simulink model "TailSitter_PX4"  (R2018b)
settings: Solver=VariableStepAuto  StartTime=0.0  StopTime=1100  RelTol=1e-3
values from neighbouring files (symbols this model uses):
  p =     [ds.mat]    (also in vxs.mat)
undefined symbols (not defined in the file or in its folder): quatnormalize
libraries: aerolibutil x24, simulink x14, sharedtransform x6, vrlib x4, sharedutil x3, simulink_extras x2, aerolibanim x1, aerolibanimutils x1
(part 3 of 3)

== matlab function TailSitter_PX4/AdHoc2 ==
  data: u_jointT input; u_omegaL output; u_omegaR output; u_deltaL output; u_deltaR output; tx input; ty input; tz input
function [u_omegaL,u_omegaR, u_deltaL,u_deltaR]  = AdHocTorques( u_jointT, tx, ty, tz)

% This is a crude/simple input/output/actuator linker.
% A pitch torque is made by moving elevons in the same direction: jointA.
% A roll torque is made by moving elevons in opposite direction: deltaA.
% A yaw torque is made by a differential thrust of the engines: deltaT.
% Power forward is given and passed straight through this function as
% jointT.

u_deltaL = 0;
u_deltaR = 0;
u_omegaL = 0;
u_omegaR = 0;



u_deltaA = -tx;
u_jointA = -ty;
u_deltaT = -tz;

u_deltaL = u_jointA - u_deltaA/2;
u_deltaR = u_jointA + u_deltaA/2;
u_omegaL = u_jointT + u_deltaT/2;
u_omegaR = u_jointT - u_deltaT/2;


end

== matlab function TailSitter_PX4/MATLAB Function3 ==
  data: v_wf input; yaw output; vr_wf input
function yaw = fcn(v_wf, vr_wf)

yawr = atan2(vr_wf(2),vr_wf(1));

if abs(atan2(sqrt(sum(v_wf(1:2).^2)),abs(v_wf(3)))) < 0.1
    yaw = yawr;
else
    yaw = atan2(v_wf(2),v_wf(1));
end

== matlab function TailSitter_PX4/TorqueTranslator ==
  data: u_jointT input; states input; wdots input; pitchoffset input; p parameter; u_omegaL output; u_omegaR output; u_deltaL output; u_deltaR output; equivalent_gains output size=[1,3]
function [u_omegaL, u_omegaR, u_deltaL, u_deltaR, equivalent_gains] = torqueConverter(u_jointT,states, wdots, pitchoffset, p)

% The reference coming in is for angular accelleration, so don't treat it
% as pure torque:
% I*wdot = tao 

%wxr = taos(1)./p.Ix; 
%wyr = taos(2)./p.Iy;
%wzr = taos(3)./p.Iz;

tx = wdots(1)*p.Ix;
ty = wdots(2)*p.Iy;
tz = wdots(3)*p.Iz;
v = states(1:3);
vx = v(1);
vy = v(2);
vz = v(3);

omegaL = states(13);
omegaR = states(14);

%init outputs
u_deltaL = 0;
u_deltaR = 0;
u_omegaL = 0;
u_omegaR = 0;


% We assume propellers always spin one way. Never reverse.
% We know wanted torque, i.e. we know wdot*Iz=taoz=p.yt*(TL-TR)=p.yt*dT
% taoz./p.yt = TL-TR = p.K_T*(omegaL^2-omegaR^2)
% taoz/(p.yt*p.K_T) = omegaL^2-omegaR^2
% we also know
%TL = JT+dT/2
%TR = JT-dt/2
% => TL-TR = dT = taoz
% if TL=p.K_T*omegaL^2 then
%omegaL=sqrt(TL/p.K_T) =>
%omegaL=sqrt( (JT+dt/2)/p.K_T )
u_omegaL2 = (u_jointT+(tz/p.yt)/2)/p.K_T ; % THese share the jointT, half each.
u_omegaR2 =  (u_jointT-(tz/p.yt)/2)/p.K_T ;
if u_omegaL2 < 0
    u_omegaL = 0;
else
    u_omegaL = sqrt(u_omegaL2);
end
if u_omegaR2 < 0
    u_omegaR = 0;
else
    u_omegaR = sqrt(u_omegaR2);
end

% Lets make a few (crude) approximations.
% - Damping due to rotational speed doesn't exist.
% - Winglets have no z-offset.
% - Wings provide no pitch moment from lift
% Then we come to these formulas for torque around each axis:
%f1 = p.yf.*(FLT+FL -FRT-FR)
%f2 = p.xf.*(FLT+FL+FRT+FR) ...
%f3 = p.yt.*(TL-TR) ...
% 
% They essentially say that aileroins are effective proportioanlly to the
% (square) of the air velocity over them.
% Lets invert that and use as our tunable gain.

% airflow in thrust wake
v_w_L = p.b_w .* omegaL; %[b_w .* omegaL; vy; vz];
v_w_R = p.b_w .* omegaR;
% AILERONS
% Lift inside wake, signs bc rotation dir of aileron
%dFT = -p.CLdelta * 0.5*p.rho * p.Saw;% * deltaL*v_w_L.^2;
 dFT = -p.CLdelta * 0.5*p.rho * p.Saw;% * deltaR*v_w_R.^2;
% Lift outside wake
dF = -sign(vx).*p.CLdelta * 0.5*p.rho*(vx.^2 + vy.^2 + vz.^2) * p.Sa;% * deltaL;

%taoy = p.xf.*(FLT+FL+FRT+FR) ...
%taoy/p.xf = FLT+FL+FRT+FR
%taoy/p.xf = dFT*deltaL*v_w_L.^2 + dFT*deltaR*v_w_R.^2 +dF*(deltaL+deltaR);
%taoy/p.xf = dFT*jointA*v_w_L.^2 + dFT*jointA*v_w_R.^2 +dF*(2*jointA);
%taoy/p.xf = jointA(dFT*v_w_L.^2 + dFT*v_w_R.^2 +dF*2);
%taoy/(p.xf*(dFT*v_w_L.^2 + dFT*v_w_R.^2 +dF*2)) = jointA;
%%%u_jointA = ty/(p.xf*(dFT*v_w_L.^2 + dFT*v_w_R.^2 +dF*2));


%taox/p.yf = (dFLT+dFL)*deltaL - (dFRT+dFR)*deltaR;
%taox/p.yf = dF(deltaL-deltaR) + dFLT*deltaL -dFRT*deltaR;
%toax/p.yf = dF(deltaL-deltaR) + dFT*(deltaL*v_w_L.^2 - deltaR*v_w_R.^2)
%toax/p.yf = -dF*dA + dFT*(deltaL*v_w_L.^2 - deltaR*v_w_R.^2)

%deltaL = JA - dA/2; % Probably bad assumption, jump to other assumptiom
%deltaR = JA + dA/2; => 
%toax/p.yf = -dF*dA + dFT*((JA-dA/2)*v_w_L.^2 - (JA+dA/2)*v_w_R.^2)
%toax/p.yf = -dF*dA + dFT*( JA*v_w_L.^2 - dA*v_w_L.^2/2 - JA*v_w_R.^2 + dA*v_w_R.^2/2)
%toax/p.yf = -dF*dA + dFT*JA(v_w_L.^2-v_w_R.^2) - ( dA*v_w_L.^2/2  - dA*v_w_R.^2/2)
%toax/p.yf - dFT*JA(v_w_L.^2-v_w_R.^2) = -dF*dA - dA*(v_w_L.^2 -v_w_R.^2)/2
%toax/p.yf - dFT*JA(v_w_L.^2-v_w_R.^2) = -dA(dF + (v_w_L.^2 -v_w_R.^2)/2)
%-(toax/p.yf - dFT*JA(v_w_L.^2-v_w_R.^2)) / (dF + (v_w_L.^2 -v_w_R.^2)/2) = dA
%u_deltaA = -(tx/p.yf - dFT*u_jointA*(v_w_L.^2-v_w_R.^2)) / (dF + (v_w_L.^2 -v_w_R.^2)/2);

%taox/p.yf = (dFLT+dFL)*deltaL - (dFRT+dFR)*deltaR;
%taox/p.yf = dF(deltaL-deltaR) + dFLT*deltaL -dFRT*deltaR;
%toax/p.yf = dF(deltaL-deltaR) + dFT*(deltaL*v_w_L.^2 - deltaR*v_w_R.^2)
%toax/p.yf = -dF*dA + dFT*(deltaL*v_w_L.^2 - deltaR*v_w_R.^2)

%deltaL = -dA/2; % Maube correct assumption?
%deltaR = +dA/2; => 
%toax/p.yf = -dF*dA + dFT*((-dA/2)*v_w_L.^2 - (+dA/2)*v_w_R.^2)
%toax/p.yf = -dF*dA + dFT*( - dA*v_w_L.^2/2   dA*v_w_R.^2/2)
%toax/p.yf = -dF*dA - ( dA*v_w_L.^2/2  - dA*v_w_R.^2/2)
%toax/p.yf = -dF*dA - dA*(v_w_L.^2 -v_w_R.^2)/2
%toax/p.yf = -dA(dF + (v_w_L.^2 -v_w_R.^2)/2)
%-(toax/p.yf) / (dF + (v_w_L.^2 -v_w_R.^2)/2) = dA
%%%u_deltaA = -(tx/p.yf) / (dF + 0*0.5*(v_w_L.^2 -v_w_R.^2));


%u_deltaA = (365.0*(3.66e97*omegaL^2*tx + 3.66e97*omegaR^2*tx - 6.17e97*omegaL^2*ty + 6.17e97*omegaR^2*ty - 1.32e91*omegaL^3*abs(omegaL) + 1.32e91*omegaR^3*abs(omegaR) - 2.53e94*omegaL^2*vx*(vx^2 + vz^2)^(1/2) + 2.53e94*omegaR^2*vx*(vx^2 + vz^2)^(1/2) - 2.59e95*omegaL^2*vz*(vx^2 + vz^2)^(1/2) + 2.59e95*omegaR^2*vz*(vx^2 + vz^2)^(1/2) + 1.32e91*omegaL*omegaR^2*abs(omegaL) - 1.32e91*omegaL^2*omegaR*abs(omegaR) + 6.36e100*tx*vx^2*sign(vx) + 6.36e100*tx*vy^2*sign(vx) + 6.36e100*tx*vz^2*sign(vx) + 2.53e95*omegaL^2*vz*cos(2.0*atan2(1.0*vz, vx))*(vx^2 + vz^2)^(1/2) - 2.53e95*omegaR^2*vz*cos(2.0*atan2(1.0*vz, vx))*(vx^2 + vz^2)^(1/2) - 1.52e95*omegaL^2*vx*sin(2.0*atan2(1.0*vz, vx))*(vx^2 + vz^2)^(1/2) + 1.52e95*omegaR^2*vx*sin(2.0*atan2(1.0*vz, vx))*(vx^2 + vz^2)^(1/2)))/(8.21e100*vx^4*sign(vx)^2 + 8.21e100*vy^4*sign(vx)^2 + 8.21e100*vz^4*sign(vx)^2 + 1.09e95*omegaL^2*omegaR^2 + 1.64e101*vx^2*vy^2*sign(vx)^2 + 1.64e101*vx^2*vz^2*sign(vx)^2 + 1.64e101*vy^2*vz^2*sign(vx)^2 + 9.45e97*omegaL^2*vx^2*sign(vx) + 9.45e97*omegaR^2*vx^2*sign(vx) + 9.45e97*omegaL^2*vy^2*sign(vx) + 9.45e97*omegaR^2*vy^2*sign(vx) + 9.45e97*omegaL^2*vz^2*sign(vx) + 9.45e97*omegaR^2*vz^2*sign(vx));
%u_jointA = -(1.46*(4.58e99*omegaR^2*tx - 4.58e99*omegaL^2*tx + 7.71e99*omegaL^2*ty + 7.71e99*omegaR^2*ty + 1.64e93*omegaL^3*abs(omegaL) + 1.64e93*omegaR^3*abs(omegaR) + 3.16e96*omegaL^2*vx*(vx^2 + vz^2)^(1/2) + 3.16e96*omegaR^2*vx*(vx^2 + vz^2)^(1/2) + 3.24e97*omegaL^2*vz*(vx^2 + vz^2)^(1/2) + 3.24e97*omegaR^2*vz*(vx^2 + vz^2)^(1/2) + 1.64e93*omegaL*omegaR^2*abs(omegaL) + 1.64e93*omegaL^2*omegaR*abs(omegaR) + 5.49e99*vx^3*sign(vx)*(vx^2 + vz^2)^(1/2) + 5.63e100*vz^3*sign(vx)*(vx^2 + vz^2)^(1/2) + 1.34e103*ty*vx^2*sign(vx) + 1.34e103*ty*vy^2*sign(vx) + 1.34e103*ty*vz^2*sign(vx) + 5.49e99*vx*vy^2*sign(vx)*(vx^2 + vz^2)^(1/2) + 5.49e99*vx*vz^2*sign(vx)*(vx^2 + vz^2)^(1/2) + 5.63e100*vx^2*vz*sign(vx)*(vx^2 + vz^2)^(1/2) + 5.63e100*vy^2*vz*sign(vx)*(vx^2 + vz^2)^(1/2) + 2.86e96*omegaL*vx^2*abs(omegaL)*sign(vx) + 2.86e96*omegaR*vx^2*abs(omegaR)*sign(vx) + 2.86e96*omegaL*vy^2*abs(omegaL)*sign(vx) + 2.86e96*omegaR*vy^2*abs(omegaR)*sign(vx) + 2.86e96*omegaL*vz^2*abs(omegaL)*sign(vx) + 2.86e96*omegaR*vz^2*abs(omegaR)*sign(vx) - 3.16e97*omegaL^2*vz*cos(2.0*atan2(1.0*vz, vx))*(vx^2 + vz^2)^(1/2) - 3.16e97*omegaR^2*vz*cos(2.0*atan2(1.0*vz, vx))*(vx^2 + vz^2)^(1/2) + 1.9e97*omegaL^2*vx*sin(2.0*atan2(1.0*vz, vx))*(vx^2 + vz^2)^(1/2) + 1.9e97*omegaR^2*vx*sin(2.0*atan2(1.0*vz, vx))*(vx^2 + vz^2)^(1/2) - 5.49e100*vz^3*cos(2.0*atan2(1.0*vz, vx))*sign(vx)*(vx^2 + vz^2)^(1/2) + 3.29e100*vx^3*sin(2.0*atan2(1.0*vz, vx))*sign(vx)*(vx^2 + vz^2)^(1/2) - 5.49e100*vx^2*vz*cos(2.0*atan2(1.0*vz, vx))*sign(vx)*(vx^2 + vz^2)^(1/2) - 5.49e100*vy^2*vz*cos(2.0*atan2(1.0*vz, vx))*sign(vx)*(vx^2 + vz^2)^(1/2) + 3.29e100*vx*vy^2*sin(2.0*atan2(1.0*vz, vx))*sign(vx)*(vx^2 + vz^2)^(1/2) + 3.29e100*vx*vz^2*sin(2.0*atan2(1.0*vz, vx))*sign(vx)*(vx^2 + vz^2)^(1/2)))/(8.21e100*vx^4*sign(vx)^2 + 8.21e100*vy^4*sign(vx)^2 + 8.21e100*vz^4*sign(vx)^2 + 1.09e95*omegaL^2*omegaR^2 + 1.64e101*vx^2*vy^2*sign(vx)^2 + 1.64e101*vx^2*vz^2*sign(vx)^2 + 1.64e101*vy^2*vz^2*sign(vx)^2 + 9.45e97*omegaL^2*vx^2*sign(vx) + 9.45e97*omegaR^2*vx^2*sign(vx) + 9.45e97*omegaL^2*vy^2*sign(vx) + 9.45e97*omegaR^2*vy^2*sign(vx) + 9.45e97*omegaL^2*vz^2*sign(vx) + 9.45e97*omegaR^2*vz^2*sign(vx));


%u_deltaL = u_jointA - u_deltaA/2;
%u_deltaR = u_jointA + u_deltaA/2;

% Below includes pitch down moment from lift
%u_deltaL = -(1.0*(0.5*ty - 0.00102*(vx^2 + vz^2)^(1/2)*(vz*(2.0*cos(2.0*atan2(1.0*vz, vx)) - 2.05) - 1.0*vx*(1.2*sin(2.0*atan2(1.0*vz, vx)) + 0.2)) + 2.13e-7*omegaL*abs(omegaL)))/(0.00209*sign(vx)*(vx^2 + vy^2 + vz^2) + 2.41e-6*omegaL^2) - (0.5*tx)/(0.00353*sign(vx)*(vx^2 + vy^2 + vz^2) + 4.06e-6*omegaL^2);
%u_deltaR =  (0.5*tx)/(0.00353*sign(vx)*(vx^2 + vy^2 + vz^2) + 4.06e-6*omegaR^2) - (1.0*(0.5*ty - 0.00102*(vx^2 + vz^2)^(1/2)*(vz*(2.0*cos(2.0*atan2(1.0*vz, vx)) - 2.05) - 1.0*vx*(1.2*sin(2.0*atan2(1.0*vz, vx)) + 0.2)) + 2.13e-7*omegaR*abs(omegaR)))/(0.00209*sign(vx)*(vx^2 + vy^2 + vz^2) + 2.41e-6*omegaR^2);

% Below only includes sensitivity from airflow % The pitch offet is our
% mechanical trim on the aircraft.
v2 = (vx^2 + vy^2 + vz^2);
omegaL_f = omegaL; %omegas_filt(1);
omegaR_f = omegaR; %omegas_filt(2);
u_deltaL = -(0.5*ty) / (0.00209*sign(vx)*v2 + 2.41e-6*omegaL_f.^2) - (0.5*tx) / (0.00353*sign(vx)*v2 + 4.06e-6*omegaL_f.^2) + pitchoffset;
u_deltaR =  (0.5*tx) / (0.00353*sign(vx)*v2 + 4.06e-6*omegaR_f.^2) - (0.5*ty) / (0.00209*sign(vx)*v2 + 2.41e-6*omegaR_f.^2) + pitchoffset;
 

% The equivalent gains are very misleading, so don't use them much.
equivalent_gains = [ (u_deltaL-u_deltaR)./tx, 0.5*(u_deltaL+u_deltaR)./ty, ...
    (u_omegaL-u_omegaR)./tz];

== matlab function TailSitter_PX4/MATLAB Function5 ==
  data: angErr input; taos output; w input; hovermode input
function taos = fcn(angErr, w, hovermode)

taos = [0;0;0];

P1_fly = 4;
P2_fly = 1.5;
cx_fly = -1;
cy_fly = 1;
cz_fly = -30;

P1_hover = 4;
P2_hover = 2.5-0.5;
cx_hover = -0.6/20;
cy_hover =  0.6;
cz_hover = -120;

if hovermode
    % Emil Fresk P2 controller
    taos = -P1_hover.*angErr - P2_hover.*w;
    % Adjustment for actuators
    taos(1) = cx_hover*taos(1);
    taos(2) = cy_hover*taos(2);
    taos(3) = cz_hover*taos(3);
else
    taos = -P1_fly.*angErr - P2_fly.*w;
    taos(1) = cx_fly*taos(1);
    taos(2) = cy_fly*taos(2);
    taos(3) = cz_fly*taos(3);
end
